simulink model "Test_Off_Grid_Inverter_Control_LC"  (R2023b)
settings: Solver=VariableStepAuto  StartTime=0.0  StopTime=5  RelTol=1e-3
InitFcn:
  | %Initialization_for_ESS_3P_2L_220kW;
  | Initialization_for_ESS_3P_2L_220kW;
values from neighbouring files (symbols this model uses):
  C_grid = 45e-6    (= 4.5e-05)    [Initialization_for_ESS_3P_2L_220kW.m]    (also in Initialization_for_Testbench.m)
  Cdc = 180e-6    (= 0.00018)    [CurrentLoop.m]    (also in Initialization_for_ESS_3P_2L_220kW.m; Initialization_for_Testbench.m)
  L_grid = 200e-6    (= 0.0002)    [Initialization_for_ESS_3P_2L_220kW.m]    (also in Initialization_for_Testbench.m)
  Ts_Control = 62.5e-6    (= 6.25e-05)    [CurrentLoop.m]    (also in Initialization_for_ESS_3P_2L_220kW.m; Initialization_for_Testbench.m = 0.0001)
  Ts_Power = 10e-7    (= 1e-06)    [Initialization_for_ESS_3P_2L_220kW.m]    (also in Initialization_for_Testbench.m)
  Udc_ref = 1500    [CurrentLoop.m]    (also in Initialization_for_ESS_3P_2L_220kW.m; Initialization_for_Testbench.m)
libraries: spsVoltageMeasurementLib x4, spsThreePhaseVIMeasurementLib x3, spsThreePhaseSeriesRLCBranchLib x2, spsThreePhaseSeriesRLCLoadLib x2, spsThreePhaseBreakerLib x2, spsTriangleGeneratorLib x1, spsDCVoltageSourceLib x1, spsSeriesRLCBranchLib x1, spsUniversalBridgeLib x1, spspowerguiLib x1
settings Model: DataDictionary=Off_Grid_Inverter_Control_LC.sldd  Creator=ZZY  LastModifiedBy=ZZY
settings DataIOCC: ReturnWorkspaceOutputs=off
settings OptimizationCC: UseDivisionForNetSlopeComputation=on

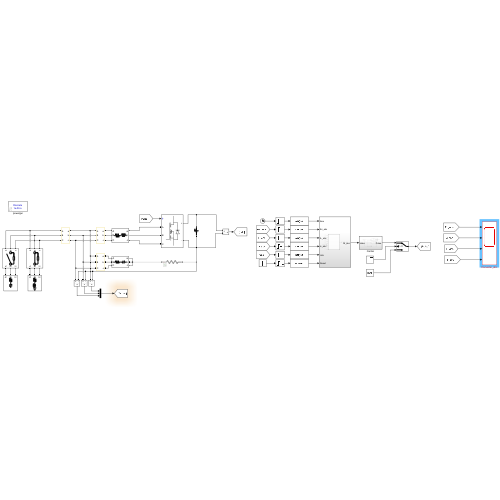
[thumbnail: Simulink's stored preview of the top-level diagram]
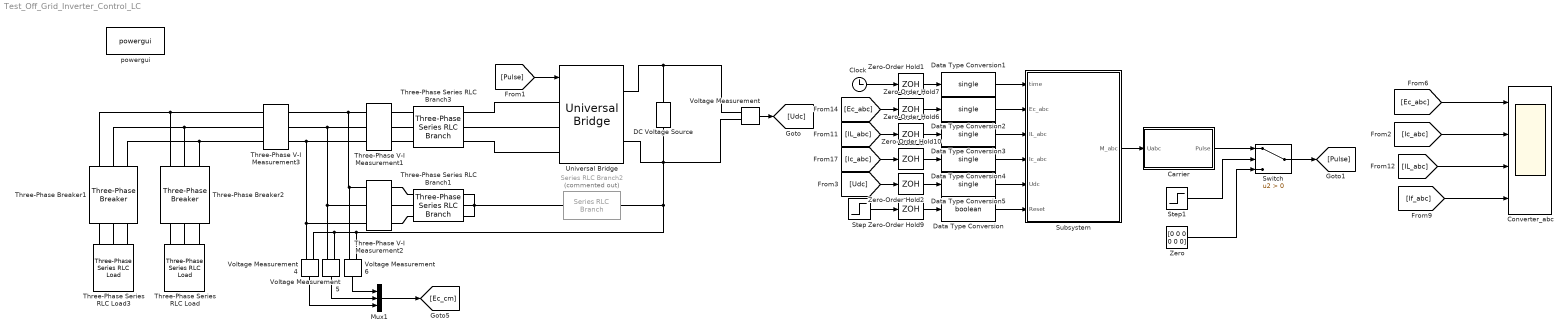
== system Test_Off_Grid_Inverter_Control_LC ==
  Carrier : Subsystem
  Clock : Clock
  Converter_abc : Scope  NumInputPorts=4
  DC Voltage Source : spsDCVoltageSourceLib/DC Voltage Source  Amplitude=Udc_ref  Measurements=None
  Data Type Conversion : DataTypeConversion  OutDataTypeStr=boolean  SaturateOnIntegerOverflow=off  RndMeth=Floor
  Data Type Conversion{1..5} (5 alike) : DataTypeConversion  OutDataTypeStr=single  SaturateOnIntegerOverflow=off  RndMeth=Floor
  Mux1 : Mux  Inputs=3
  Series RLC Branch2 : spsSeriesRLCBranchLib/Series RLC Branch  Commented=on  LConnTagsString=__new0  RConnTagsString=__new0  BranchType=R  Resistance=1e-6  Inductance=1e-8  SetiL0=off  InitialCurrent=0  Capacitance=Cdc  Setx0=on  InitialVoltage=750  Measurements=Branch voltage
  Step : Step  Time=0.2  OutDataTypeStr=Inherit: Inherit via back propagation  SampleTime=Ts_Control
  Step1 : Step  Time=0.2  OutDataTypeStr=Inherit: Inherit via back propagation
  Subsystem : Subsystem
  Switch : Switch  Criteria=u2 > Threshold  SaturateOnIntegerOverflow=off  InputSameDT=off
  Three-Phase Series RLC Branch1 : spsThreePhaseSeriesRLCBranchLib/Three-Phase Series RLC Branch  LConnTagsString=A|B|C  RConnTagsString=A|B|C  BranchType=RC  Resistance=10e-3  Inductance=1e-3  Capacitance=C_grid*0.8  Measurements=None
  Three-Phase Series RLC Branch3 : spsThreePhaseSeriesRLCBranchLib/Three-Phase Series RLC Branch  LConnTagsString=A|B|C  RConnTagsString=A|B|C  BranchType=RL  Resistance=1e-6  Inductance=L_grid*5  Capacitance=1e-6  Measurements=None
  Three-Phase Series RLC Load : spsThreePhaseSeriesRLCLoadLib/Three-Phase Series RLC Load  LConnTagsString=A|B|C  Configuration=Y (grounded)  NominalVoltage=690  Vabc=[1e3 1e3 1e3]  Vabcp=[1e3 1e3 1e3]  NominalFrequency=50  UnbalancedPower=off  ActivePower=20e3  InductivePower=10e3  CapacitivePower=0  Pabc=[10e3 9e3 11e3]  QLabc=[100 90 110]  QCabc=[100 90 110]  Pabcp=[10e3 9e3 11e3]  QLabcp=[100 90 110]  QCabcp=[100 90 110]  Measurements=None  LoadType=constant Z
  Three-Phase Series RLC Load3 : spsThreePhaseSeriesRLCLoadLib/Three-Phase Series RLC Load  LConnTagsString=A|B|C  Configuration=Delta  NominalVoltage=690  Vabc=[1e3 1e3 1e3]  Vabcp=[1e3 1e3 1e3]  NominalFrequency=50  UnbalancedPower=off  ActivePower=100e3  InductivePower=0  CapacitivePower=10e3  Pabc=[10e3 9e3 11e3]  QLabc=[100 90 110]  QCabc=[100 90 110]  Pabcp=[10e3 9e3 11e3]  QLabcp=[100 90 110]  QCabcp=[100 90 110]  Measurements=None  LoadType=constant Z
  Three-Phase V-I Measurement1 : spsThreePhaseVIMeasurementLib/Three-Phase V-I Measurement  VoltageMeasurement=no  SetLabelV=on  LabelV=Ec_abc  Vpu=off  VpuLL=off  CurrentMeasurement=yes  SetLabelI=on  LabelI=IL_abc  Ipu=off  Pbase=100e6  Vbase=500e3  OutputType=Complex  PhasorSimulation=off  PSBequivalent=0
  Three-Phase V-I Measurement2 : spsThreePhaseVIMeasurementLib/Three-Phase V-I Measurement  VoltageMeasurement=no  SetLabelV=off  LabelV=Ec_abc  Vpu=off  VpuLL=off  CurrentMeasurement=yes  SetLabelI=on  LabelI=If_abc  Ipu=off  Pbase=100e6  Vbase=500e3  OutputType=Complex  PhasorSimulation=off  PSBequivalent=0
  Three-Phase V-I Measurement3 : spsThreePhaseVIMeasurementLib/Three-Phase V-I Measurement  VoltageMeasurement=phase-to-ground  SetLabelV=on  LabelV=Ec_abc  Vpu=off  VpuLL=off  CurrentMeasurement=yes  SetLabelI=on  LabelI=Ic_abc  Ipu=off  Pbase=100e6  Vbase=500e3  OutputType=Complex  PhasorSimulation=off  PSBequivalent=0
  Three-Phase Breaker1 : spsThreePhaseBreakerLib/Three-Phase Breaker  InitialState=open  SwitchA=on  SwitchB=on  SwitchC=on  SwitchTimes="[2  6]"  External=off  BreakerResistance=0.01  SnubberResistance=1e6  SnubberCapacitance=inf  Measurements=None
  Three-Phase Breaker2 : spsThreePhaseBreakerLib/Three-Phase Breaker  InitialState=closed  SwitchA=on  SwitchB=on  SwitchC=on  SwitchTimes="[4  7]"  External=off  BreakerResistance=0.01  SnubberResistance=1e6  SnubberCapacitance=inf  Measurements=None
  Universal Bridge : spsUniversalBridgeLib/Universal Bridge  Arms=3  SnubberResistance=1e5  SnubberCapacitance=inf  Device=MOSFET / Diodes  Ron=1e-3  Lon=0  ForwardVoltages="[  0  0  ]"  ForwardVoltage=0  GTOparameters=[ 10e-6 , 20e-6 ]  IGBTparameters=[ 1e-6 , 2e-6 ]  Measurements=None  Measurements_2=None  converterType=Rectifier
  Voltage Measurement{,4..6} (4 alike) : spsVoltageMeasurementLib/Voltage Measurement  PhasorSimulation=off  OutputType=Complex  PSBequivalent=0
  Zero : Constant  Value=[0 0 0 0 0 0]  OutDataTypeStr=Inherit: Inherit via back propagation
  Zero-Order Hold{1..2,6..7,9..10} (6 alike) : ZeroOrderHold  SampleTime=Ts_Control
  powergui : spspowerguiLib/powergui  Priority=1  SimulationMode=Discrete  SampleTime=Ts_Power  frequency=60  Iterations=50  frequencyindice=0  Pbase=100e6  ErrMax=1e-4  UnitsV=kV  UnitsW=MW  buscounter=0  FunctionMessages=off  echomessages=off  EnableUseOfTLC=off  CurrentSourceSwitches=off  DisableSnubberDevices=off  DisableRonSwitches=off  DisableVfSwitches=off  DisplayEquations=off  AutomaticDiscreteSolvers=off  SolverType=Tustin/Backward Euler (TBE)  Interpol=off  ExternalGateDelay=off  methode=off  Ts=100  x0status=blocks  SPID=on  SwTol=0  HookPort=off  NonlinearTolerance=1e-4  nMaxIteration=100  ContinueOnMaxIteration=off  RestoreLinks=warning  ResistiveCurrentMeasurement=off  Frange=[0:2:500]  Ylog=off  Xlog=on  ShowGrid=off  save=off  variable=ZData  structure=CHB_abc  ZoomFFT=off  StartTime=1.4  cycles=5  DisplayStyle=1  fundamental=50  FreqAxis=off  MaxFrequency=30000  frequencyindicesteady=1  RmsSteady=1  display=off
  wires:
  [Ec_abc] -> Converter_abc/1
  [Ic_abc] -> Converter_abc/2
  [Pulse] -> Universal Bridge/1
  [Ec_abc] -> Zero-Order Hold7/1
  [IL_abc] -> Zero-Order Hold6/1
  Step/1 -> Zero-Order Hold9/1
  Switch/1 -> [Pulse]
  Carrier/1(Pulse) -> Switch/1
  Zero/1 -> Switch/3
  Data Type Conversion/1 -> Subsystem/6(Reset)
  Zero-Order Hold9/1 -> Data Type Conversion/1
  Step1/1 -> Switch/2
  Zero-Order Hold6/1 -> Data Type Conversion3/1
  Zero-Order Hold7/1 -> Data Type Conversion2/1
  [If_abc] -> Converter_abc/4
  [Ic_abc] -> Zero-Order Hold10/1
  Zero-Order Hold10/1 -> Data Type Conversion4/1
  [IL_abc] -> Converter_abc/3
  Voltage Measurement4/1 -> Mux1/3
  Mux1/1 -> [Ec_cm]
  Voltage Measurement6/1 -> Mux1/1
  Voltage Measurement5/1 -> Mux1/2
  Subsystem/1(M_abc) -> Carrier/1(Uabc)
  Clock/1 -> Zero-Order Hold1/1
  Zero-Order Hold1/1 -> Data Type Conversion1/1
  Zero-Order Hold2/1 -> Data Type Conversion5/1
  [Udc] -> Zero-Order Hold2/1
  Data Type Conversion1/1 -> Subsystem/1(time)
  Voltage Measurement/1 -> [Udc]
  Data Type Conversion2/1 -> Subsystem/2(Ec_abc)
  Data Type Conversion3/1 -> Subsystem/3(IL_abc)
  Data Type Conversion4/1 -> Subsystem/4(Ic_abc)
  Data Type Conversion5/1 -> Subsystem/5(Udc)
  connections:
  Three-Phase V-I Measurement1/LConn1 -- Three-Phase V-I Measurement2/LConn1 -- Voltage Measurement6/LConn1 -- Three-Phase V-I Measurement3/RConn1
  Three-Phase V-I Measurement1/LConn2 -- Three-Phase V-I Measurement2/LConn2 -- Voltage Measurement5/LConn1 -- Three-Phase V-I Measurement3/RConn2
  Three-Phase V-I Measurement1/LConn3 -- Three-Phase V-I Measurement2/LConn3 -- Voltage Measurement4/LConn1 -- Three-Phase V-I Measurement3/RConn3
  Voltage Measurement/LConn1 -- DC Voltage Source/RConn1 -- Universal Bridge/RConn1
  Three-Phase Series RLC Load3/LConn1 -- Three-Phase Breaker1/LConn1
  Three-Phase Series RLC Load3/LConn2 -- Three-Phase Breaker1/LConn2
  Three-Phase Series RLC Load3/LConn3 -- Three-Phase Breaker1/LConn3
  Three-Phase V-I Measurement1/RConn1 -- Three-Phase Series RLC Branch3/LConn1
  Three-Phase V-I Measurement1/RConn2 -- Three-Phase Series RLC Branch3/LConn2
  Three-Phase V-I Measurement1/RConn3 -- Three-Phase Series RLC Branch3/LConn3
  Three-Phase Breaker2/LConn1 -- Three-Phase Series RLC Load/LConn1
  Three-Phase Breaker2/LConn2 -- Three-Phase Series RLC Load/LConn2
  Three-Phase Breaker2/LConn3 -- Three-Phase Series RLC Load/LConn3
  Three-Phase Series RLC Branch1/LConn2 -- Three-Phase V-I Measurement2/RConn2
  Three-Phase V-I Measurement2/RConn1 -- Three-Phase Series RLC Branch1/LConn1
  Three-Phase V-I Measurement2/RConn3 -- Three-Phase Series RLC Branch1/LConn3
  Three-Phase Series RLC Branch1/RConn1 -- Series RLC Branch2/LConn1 -- Three-Phase Series RLC Branch1/RConn2 -- Three-Phase Series RLC Branch1/RConn3
  Three-Phase Breaker2/RConn1 -- Three-Phase Breaker1/RConn1 -- Three-Phase V-I Measurement3/LConn1
  Three-Phase Breaker2/RConn2 -- Three-Phase V-I Measurement3/LConn2 -- Three-Phase Breaker1/RConn2
  Three-Phase Breaker2/RConn3 -- Three-Phase V-I Measurement3/LConn3 -- Three-Phase Breaker1/RConn3
  Three-Phase Series RLC Branch3/RConn2 -- Universal Bridge/LConn2
  Universal Bridge/LConn1 -- Three-Phase Series RLC Branch3/RConn1
  Three-Phase Series RLC Branch3/RConn3 -- Universal Bridge/LConn3
  Voltage Measurement4/LConn2 -- Voltage Measurement5/LConn2 -- Voltage Measurement6/LConn2 -- Series RLC Branch2/RConn1 -- Voltage Measurement/LConn2 -- Universal Bridge/RConn2 -- DC Voltage Source/LConn1

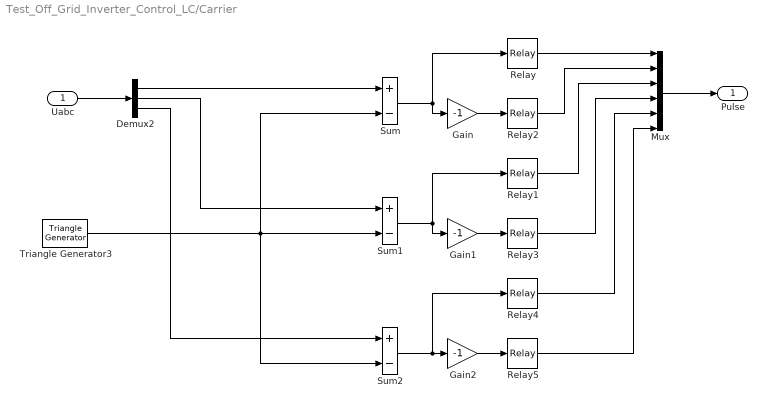
== system Test_Off_Grid_Inverter_Control_LC/Carrier ==
  Uabc : Inport
  Demux2 : Demux  Outputs=3
  Gain : Gain  Gain=-1
  Gain1 : Gain  Gain=-1
  Gain2 : Gain  Gain=-1
  Mux : Mux  Inputs=6
  Relay{,1..5} (6 alike) : Relay  OffSwitchValue=-eps
  Sum : Sum  Inputs=+-
  Sum1 : Sum  Inputs=+-
  Sum2 : Sum  Inputs=+-
  Triangle Generator3 : spsTriangleGeneratorLib/Triangle Generator  Freq=16000  Phase=180  Ts=1e-6
  Pulse : Outport
  wires:
  Mux/1 -> Pulse/1
  Gain/1 -> Relay2/1
  Sum/1 -> Relay/1, Gain/1
  Triangle Generator3/1 -> Sum2/2, Sum/2, Sum1/2
  Uabc/1 -> Demux2/1
  Demux2/1 -> Sum/1
  Relay/1 -> Mux/1
  Relay2/1 -> Mux/2
  Relay1/1 -> Mux/3
  Relay3/1 -> Mux/4
  Gain1/1 -> Relay3/1
  Demux2/2 -> Sum1/1
  Sum1/1 -> Relay1/1, Gain1/1
  Relay5/1 -> Mux/6
  Demux2/3 -> Sum2/1
  Gain2/1 -> Relay5/1
  Sum2/1 -> Relay4/1, Gain2/1
  Relay4/1 -> Mux/5

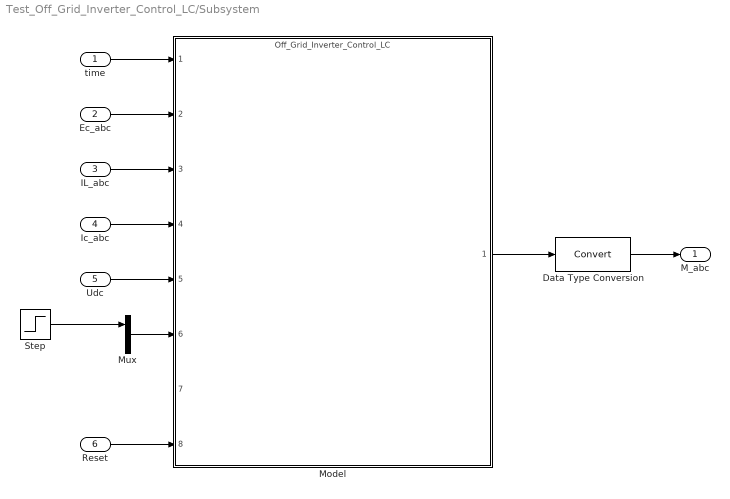
== system Test_Off_Grid_Inverter_Control_LC/Subsystem ==
  time : Inport  OutDataTypeStr=single
  Ec_abc : Inport  Port=2
  IL_abc : Inport  Port=3  OutDataTypeStr=single
  Ic_abc : Inport  Port=4  OutDataTypeStr=single
  Udc : Inport  Port=5  OutDataTypeStr=single
  Reset : Inport  Port=6  OutDataTypeStr=boolean
  Data Type Conversion : DataTypeConversion  SaturateOnIntegerOverflow=off  RndMeth=Floor
  Model : ModelReference  ModelNameDialog=Off_Grid_Inverter_Control_LC.slx  SimulationMode=Normal  ModelReferenceVersion=1.125
  Mux : Mux  Inputs=2
  Step : Step  Time=2.5  Before=1  After=0.8  OutDataTypeStr=single
  M_abc : Outport  OutDataTypeStr=single
  wires:
  Model/1 -> Data Type Conversion/1
  time/1 -> Model/1
  IL_abc/1 -> Model/3
  Ec_abc/1 -> Model/2
  Ic_abc/1 -> Model/4
  Udc/1 -> Model/5
  Reset/1 -> Model/8
  Mux/1 -> Model/6
  Step/1 -> Mux/1
  Data Type Conversion/1 -> M_abc/1
